simulink model "XYGraph"  (R2023a)
settings: Solver=ode4  StartTime=0.0  StopTime=8  FixedStep=T/j  MaxStep=8/800  RelTol=1e-4
values from neighbouring files (symbols this model uses):
  i = 12    [model.m]
  Jv = 0.006    [model.m]
  K = [ x(1:j, 1), y(1:j, 1) ]    [model.m]
  w = 2*pi/i .* v    [model.m]
settings Model: Creator=ПК  LastModifiedBy=ПК

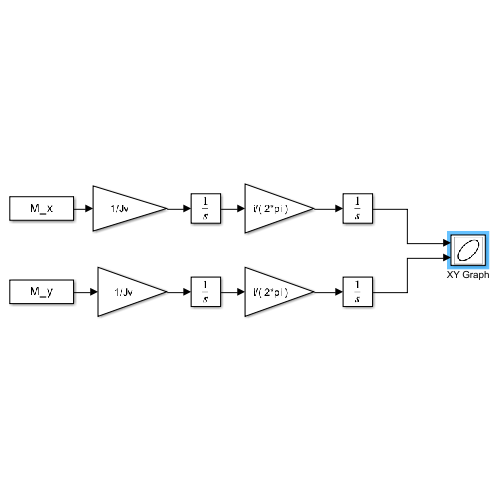
[thumbnail: Simulink's stored preview of the top-level diagram]
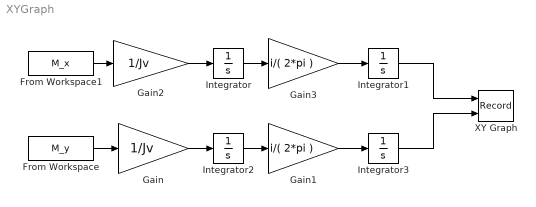
== system XYGraph ==
  From Workspace : FromWorkspace  VariableName=M_y  OutputAfterFinalValue=Setting to zero
  From Workspace1 : FromWorkspace  VariableName=M_x  OutputAfterFinalValue=Setting to zero
  Gain : Gain  Gain=1/Jv
  Gain1 : Gain  Gain=i/( 2*pi )
  Gain2 : Gain  Gain=1/Jv
  Gain3 : Gain  Gain=i/( 2*pi )
  Integrator : Integrator  InitialCondition=w(1,1)
  Integrator1 : Integrator  InitialCondition=K(1,1)
  Integrator2 : Integrator  InitialCondition=w(1,2)
  Integrator3 : Integrator  InitialCondition=K(1,2)
  XY Graph : Record  FileSettingsInternal="{\"entries\":[{\"content\":{\"excelSettings\":{\"content\":{},\"type\":\"Streamout.ExcelSettings\"}},\"type\":\"Streamout.FileSettingStorage\",\"uuid\":\"261fd0b0-1443-4a9c-a620-44da16cb5535\"}],\"packageUris\":[\"http://schema.mathworks.com/mf0/streamout_blocks/R2020a\"],\"version\":\"1.0\"}"  Layout=[1 1]  SignalsInternal="{\"entries\":[{\"content\":{\"signals\":[{\"content\":{\"blockPath\":[\"XYGraph/XY Graph\"],\"dimensions\":[1],\"domain\":\"XYGraph/XY Graph\",\"lineColor\":\"#a2142f\",\"plots\":[1],\"port\":1,\"sid\":[\"\"],\"signalID\":899,\"signalName\":\"Integrator1\"},\"type\":\"RecordBlkView.Signal\",\"uuid\":\"9aa71548-d389-48e3-be09-6169f25a676e\"},{\"content\":{\"blockPath\":[\"XYGraph/XY Graph\"],\"dimensions\":[1],\"domain\":\"XYGraph/XY Graph\",\"lineColor\":\"#139fff\",\"plots\":[1],\"port\":2,\"sid\":[\"\"],\"signalID\":903,\"signalName\":\"Integrator3\"},\"type\":\"RecordBlkView.Signal\",\"uuid\":\"20079876-d436-4b03-a541-034f356b9d9e\"}]},\"type\":\"RecordBlkView.InputSignals\",\"uuid\":\"509e5755-baf8-4413-a385-71f84f6222b2\"}],\"packageUris\":[\"http://schema.mathworks.com/mf0/streamout_blocks/R2020a\"],\"version\":\"1.0\"}"  VisualizationBindings="{\"xyplotplugin\":{\"info\":[{\"series\":[{\"bindingParametersList\":[{\"parameter\":\"X-Axis\",\"signalID\":899,\"signalName\":\"Integrator1\"},{\"parameter\":\"Y-Axis\",\"signalID\":903,\"signalName\":\"Integrator3\"}],\"seriesID\":18242}],\"subplotID\":1}]}}"  CompatibilityTag=XY
  wires:
  Integrator2/1 -> Gain1/1
  Integrator1/1 -> XY Graph/1
  From Workspace/1 -> Gain/1
  Gain/1 -> Integrator2/1
  From Workspace1/1 -> Gain2/1
  Gain2/1 -> Integrator/1
  Integrator/1 -> Gain3/1
  Gain3/1 -> Integrator1/1
  Gain1/1 -> Integrator3/1
  Integrator3/1 -> XY Graph/2
